simulink model "Observador_continuo"  (R2024a)
settings: Solver=VariableStepAuto  StartTime=0.0  StopTime=15  RelTol=1e-3
undefined symbols (not defined in the file): Aa, Bb, C, l, theta_ref
settings Model: Creator=alfar  LastModifiedBy=alfar

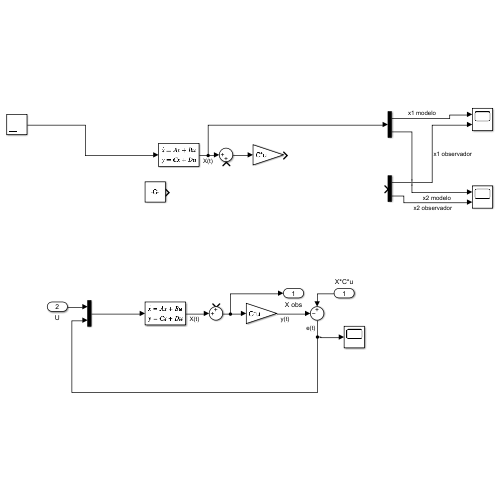
[thumbnail: Simulink's stored preview of the top-level diagram]
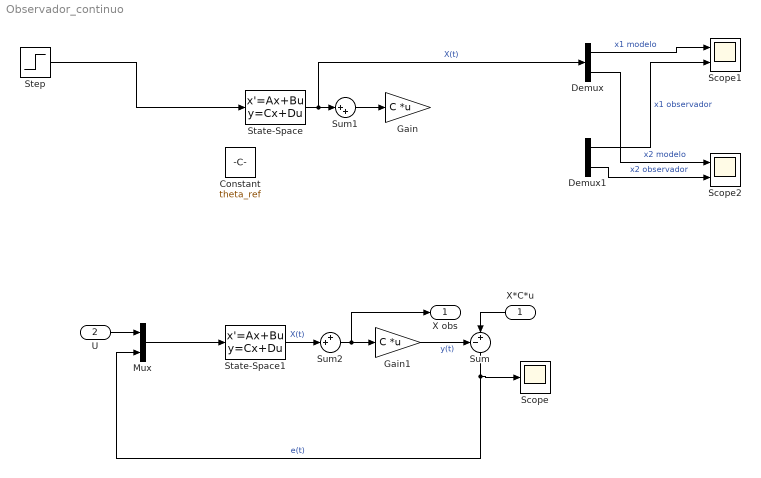
== system Observador_continuo ==
  X*C*u : Inport
  U : Inport  Port=2
  Constant : Constant  Value=theta_ref
  Demux : Demux  Outputs=2
  Demux1 : Demux  Outputs=2
  Gain : Gain  Gain=C  Multiplication=Matrix(K*u)
  Gain1 : Gain  Gain=C  Multiplication=Matrix(K*u)
  Mux : Mux  Inputs=2
  Scope : Scope
  Scope1 : Scope  NumInputPorts=2
  Scope2 : Scope  NumInputPorts=2
  State-Space : StateSpace  A=Aa  B=Bb  C=eye(2)  D=zeros(2,1)  InitialCondition=0
  State-Space1 : StateSpace  A=Aa  B=[Bb l']  C=eye(2)  D=zeros(2,2)  InitialCondition=0
  Step : Step  SampleTime=0
  Sum : Sum  Inputs=-+|
  Sum1 : Sum  Inputs=|++
  Sum2 : Sum  Inputs=++|
  X obs : Outport
  wires:
  State-Space/1 -> Sum1/1, Demux/1  "X(t)"
  Gain1/1 -> Sum/1  "y(t)"
  Sum/1 -> Scope/1, Mux/2  "e(t)"
  Mux/1 -> State-Space1/1
  Demux1/2 -> Scope2/2  "x2 observador"
  Demux1/1 -> Scope1/2  "x1 observador"
  Demux/2 -> Scope2/1  "x2 modelo"
  Demux/1 -> Scope1/1  "x1 modelo"
  Step/1 -> State-Space/1
  Sum1/1 -> Gain/1
  State-Space1/1 -> Sum2/2  "X(t)"
  Sum2/1 -> X obs/1, Gain1/1
  X*C*u/1 -> Sum/2
  U/1 -> Mux/1
